simulink model "Comparation_L_and_NL_Lat"  (R2025b)
settings: Solver=ode4  StartTime=0.0  StopTime=10  FixedStep=1/10  RelTol=1e-3
values from neighbouring files (symbols this model uses):
  sys_lat = ss(A_lat, B_lat, C_lat, D_lat,      'StateName',{'beta';'p';'r';'phi';'psi'},      'InputName',{'aileron';'rudder'},      'OutputName',{'beta';'p';'r';'phi';'psi'})    [MATRIZES_DH.m]    (also in modelo_linear_DH.m = ss(A_lat, B_lat, C_lat, D_lat,      'StateName', {'beta'; 'p)
  Ue = [0.283590235022 0.133002178957 0 0 0 0 0]'    [MATRIZES_DH.m]
undefined symbols (not defined in the file or in its folder): sigbuilder_block
settings Model: Creator=anade  LastModifiedBy=mirko

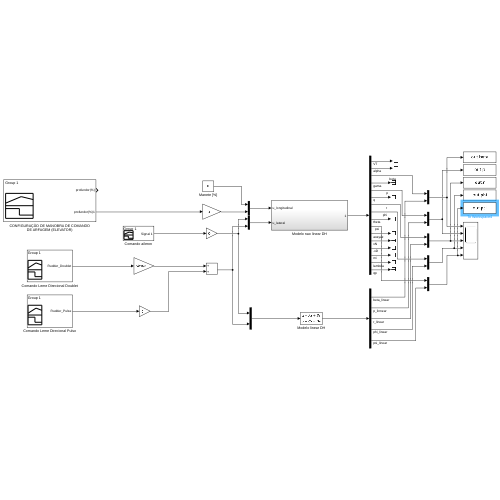
[thumbnail: Simulink's stored preview of the top-level diagram]
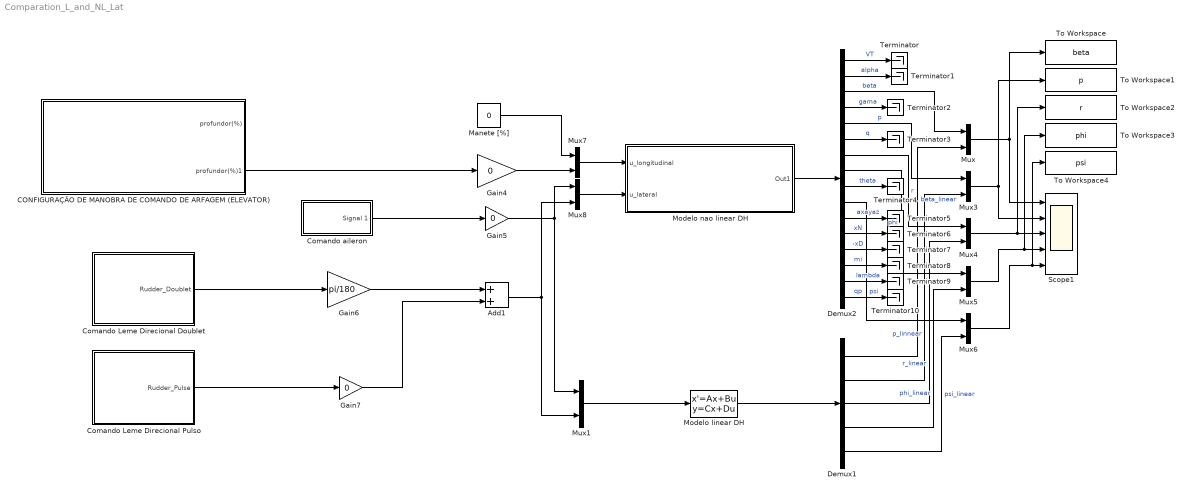
== system Comparation_L_and_NL_Lat ==
  Add1 : Sum
  CONFIGURAÇÃO DE MANOBRA DE COMANDO DE ARFAGEM (ELEVATOR) : Subsystem  Tag=STV Subsys  LoadFcn=sigbuilder_block('load');  StartFcn=sigbuilder_block('start');  StopFcn=sigbuilder_block('stop');  ClipboardFcn=sigbuilder_block('clipboard');  mask(Sigbuilder block){tuvar=[0:10]}
      mask help: Simulink:masks:SigbuilderBlock_MD
      mask init:
      | if ~strcmp(get_param(bdroot(gcbh),'SimulationStatus'),'stopped') tuvar = sigbuilder_block('maskInit'); end
      settings: CopyFcn=sigbuilder_block('copy');  DeleteFcn=sigbuilder_block('delete');  ModelCloseFcn=sigbuilder_block('modelClose');  PreSaveFcn=sigbuilder_block('preSave');  PauseFcn=sigbuilder_block('pause');  ContinueFcn=sigbuilder_block('continue');  NameChangeFcn=sigbuilder_block('namechange');  OpenFcn=sigbuilder_block('open',[437.6 199.2 550.4 400 ]);  CloseFcn=sigbuilder_block('close');
      mask Display: plot(0, 0, 100, 100,[2, 2, 32, 32, 2], [68, 8, 8, 68, 68],[32, 2], [38, 38], [32, 19, 2],[53, 60, 44], [32, 17, 17, 2],[16, 16, 31, 31]);txt = getActiveGroup(gcbh);text(2, 100, txt,'verticalAlignment', 'top');
  Comando Leme Direcional Doublet : Subsystem  Tag=STV Subsys  LoadFcn=sigbuilder_block('load');  StartFcn=sigbuilder_block('start');  StopFcn=sigbuilder_block('stop');  ClipboardFcn=sigbuilder_block('clipboard');  mask(Sigbuilder block){tuvar=[0:10]}
      mask help: Simulink:masks:SigbuilderBlock_MD
      mask init:
      | if ~strcmp(get_param(bdroot(gcbh),'SimulationStatus'),'stopped') tuvar = sigbuilder_block('maskInit'); end
      settings: CopyFcn=sigbuilder_block('copy');  DeleteFcn=sigbuilder_block('delete');  ModelCloseFcn=sigbuilder_block('modelClose');  PreSaveFcn=sigbuilder_block('preSave');  PauseFcn=sigbuilder_block('pause');  ContinueFcn=sigbuilder_block('continue');  NameChangeFcn=sigbuilder_block('namechange');  OpenFcn=sigbuilder_block('open',[316.5 171.75 805.5 485.25 ]);  CloseFcn=sigbuilder_block('close');
      mask Display: plot(0, 0, 100, 100,[2, 2, 32, 32, 2], [68, 8, 8, 68, 68],[32, 2], [38, 38], [32, 19, 2],[53, 60, 44], [32, 17, 17, 2],[16, 16, 31, 31]);txt = getActiveGroup(gcbh);text(2, 100, txt,'verticalAlignment', 'top');
  Comando Leme Direcional Pulso : Subsystem  Tag=STV Subsys  LoadFcn=sigbuilder_block('load');  StartFcn=sigbuilder_block('start');  StopFcn=sigbuilder_block('stop');  ClipboardFcn=sigbuilder_block('clipboard');  mask(Sigbuilder block){tuvar=[0:10]}
      mask help: Simulink:masks:SigbuilderBlock_MD
      mask init:
      | if ~strcmp(get_param(bdroot(gcbh),'SimulationStatus'),'stopped') tuvar = sigbuilder_block('maskInit'); end
      settings: CopyFcn=sigbuilder_block('copy');  DeleteFcn=sigbuilder_block('delete');  ModelCloseFcn=sigbuilder_block('modelClose');  PreSaveFcn=sigbuilder_block('preSave');  PauseFcn=sigbuilder_block('pause');  ContinueFcn=sigbuilder_block('continue');  NameChangeFcn=sigbuilder_block('namechange');  OpenFcn=sigbuilder_block('open',[463.8 78 543 376.2 ]);  CloseFcn=sigbuilder_block('close');
      mask Display: plot(0, 0, 100, 100,[2, 2, 32, 32, 2], [68, 8, 8, 68, 68],[32, 2], [38, 38], [32, 19, 2],[53, 60, 44], [32, 17, 17, 2],[16, 16, 31, 31]);txt = getActiveGroup(gcbh);text(2, 100, txt,'verticalAlignment', 'top');
  Comando aileron : Subsystem  Tag=STV Subsys  LoadFcn=sigbuilder_block('load');  StartFcn=sigbuilder_block('start');  StopFcn=sigbuilder_block('stop');  ClipboardFcn=sigbuilder_block('clipboard');  mask(Sigbuilder block){tuvar=[0:10]}
      mask help: Simulink:masks:SigbuilderBlock_MD
      mask init:
      | if ~strcmp(get_param(bdroot(gcbh),'SimulationStatus'),'stopped') tuvar = sigbuilder_block('maskInit'); end
      settings: CopyFcn=sigbuilder_block('copy');  DeleteFcn=sigbuilder_block('delete');  ModelCloseFcn=sigbuilder_block('modelClose');  PreSaveFcn=sigbuilder_block('preSave');  PauseFcn=sigbuilder_block('pause');  ContinueFcn=sigbuilder_block('continue');  NameChangeFcn=sigbuilder_block('namechange');  OpenFcn=sigbuilder_block('open',[6.75 6.75 1134.75 568.5 ]);  CloseFcn=sigbuilder_block('close');
      mask Display: plot(0, 0, 100, 100,[2, 2, 32, 32, 2], [68, 8, 8, 68, 68],[32, 2], [38, 38], [32, 19, 2],[53, 60, 44], [32, 17, 17, 2],[16, 16, 31, 31]);txt = getActiveGroup(gcbh);text(2, 100, txt,'verticalAlignment', 'top');
  Demux1 : Demux  Outputs=5
  Demux2 : Demux  Outputs=16
  Gain4 : Gain  Gain=0  OutDataTypeStr=double
  Gain5 : Gain  Gain=0
  Gain6 : Gain  Gain=pi/180
  Gain7 : Gain  Gain=0
  Manete [%] : Constant  Value=0
  Modelo linear DH : StateSpace  A=sys_lat.A  B=sys_lat.B  C=sys_lat.C  D=sys_lat.D  InitialCondition=[0 0 0 0 0]
  Modelo nao linear DH : Subsystem
  Mux{,1,3..8} (8 alike) : Mux  Inputs=2
  Scope1 : Scope  NumInputPorts=5
      settings: ActiveDisplayYMinimum=-4.5855532586935484  ActiveDisplayYMaximum=3.8994861451279332
  Terminator{,1..10} (11 alike) : Terminator
  To Workspace : ToWorkspace  VariableName=beta  SaveFormat=Structure With Time  SampleTime=-1
  To Workspace1 : ToWorkspace  VariableName=p  SaveFormat=Structure With Time  SampleTime=-1
  To Workspace2 : ToWorkspace  VariableName=r  SaveFormat=Structure With Time  SampleTime=-1
  To Workspace3 : ToWorkspace  VariableName=phi  SaveFormat=Structure With Time  SampleTime=-1
  To Workspace4 : ToWorkspace  VariableName=psi  SaveFormat=Structure With Time  SampleTime=-1
  wires:
  Mux1/1 -> Modelo linear DH/1
  Modelo linear DH/1 -> Demux1/1
  Mux/1 -> To Workspace/1, Scope1/1
  Demux1/2 -> Mux3/2  "p_linnear"
  Demux1/3 -> Mux4/2  "r_linear"
  Demux1/4 -> Mux5/2  "phi_linear"
  Demux1/5 -> Mux6/2  "psi_linear"
  Mux3/1 -> To Workspace1/1, Scope1/2
  Mux4/1 -> Scope1/3, To Workspace2/1
  Mux5/1 -> To Workspace3/1, Scope1/4
  Mux6/1 -> To Workspace4/1, Scope1/5
  Demux1/1 -> Mux/2  "beta_linear"
  Mux7/1 -> Modelo nao linear DH/1(u_longitudinal)
  Gain7/1 -> Add1/2
  Comando Leme Direcional Pulso/1(Rudder_Pulse) -> Gain7/1
  Modelo nao linear DH/1(Out1) -> Demux2/1
  Gain5/1 -> Mux8/1, Mux1/1
  Comando Leme Direcional Doublet/1(Rudder_Doublet) -> Gain6/1
  Demux2/3 -> Mux/1  "beta"
  Gain4/1 -> Mux7/2
  Comando aileron/1(Signal 1) -> Gain5/1
  Demux2/10 -> Mux6/1  "psi"
  Demux2/5 -> Mux3/1  "p"
  Gain6/1 -> Add1/1
  Demux2/8 -> Mux5/1  "phi"
  CONFIGURAÇÃO DE MANOBRA DE COMANDO DE ARFAGEM (ELEVATOR)/2(profundor(%)1) -> Gain4/1
  Mux8/1 -> Modelo nao linear DH/2(u_lateral)
  Demux2/7 -> Mux4/1  "r"
  Add1/1 -> Mux8/2, Mux1/2
  Manete [%]/1 -> Mux7/1
  Demux2/1 -> Terminator/1  "VT"
  Demux2/2 -> Terminator1/1  "alpha"
  Demux2/4 -> Terminator2/1  "gama"
  Demux2/6 -> Terminator3/1  "q"
  Demux2/9 -> Terminator4/1  "theta"
  Demux2/11 -> Terminator5/1  "axayaz"
  Demux2/12 -> Terminator6/1  "xN"
  Demux2/13 -> Terminator7/1  "-xD"
  Demux2/14 -> Terminator8/1  "mi"
  Demux2/15 -> Terminator9/1  "lambda"
  Demux2/16 -> Terminator10/1  "qp"

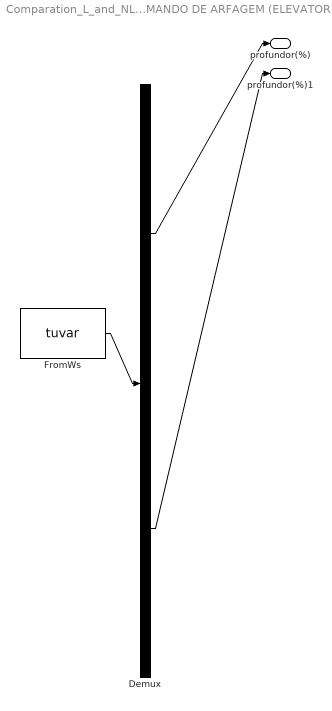
== system Comparation_L_and_NL_Lat/CONFIGURAÇÃO DE MANOBRA DE COMANDO DE ARFAGEM (ELEVATOR) ==
  Demux : Demux  Tag=STV Demux  Outputs=2
      settings: DisplayOption=none
  FromWs : FromWorkspace  Tag=STV FromWs  VariableName=tuvar
      SigBuilderData=|
      | common.afterFinalStr = 'Extrapolate'
      | common.sampleTime = '0'
      | dataSet.timeRange = [0 100]
      | dataSet.name = 'Group 1'
      | sbobj.Groups.Name = 'Group 1'
      | sbobj.Groups.Signals(1).Name = 'profundor(%)'
      | sbobj.Groups.Signals(1).XData = [0 0.1 0.2 0.3 0.4 0.5 0.6 0.7 0.8 0.9 1 1.1 1.2 1.3 1.4 1.5 1.6 1.7 1.8 1.9 2 2.1 2.2 2.3 2.4 2.5 2.6 2.7 2.8 2.9 3 3.1 3.2 3.3 3.4 3.5 3.6 3.7 3.8 3.9 4 4.1 4.2 4.3 4.4 4.5 4.6 4.7 4.8 4.9 5 5.1 5.2 5.3 5.4 5.5 5.6 5.7 5.8 5.9 6 6.1 6.2 6.3 6.4 6.5 6.6 6.7 6.8 6.9 7 7.1 7.2 7.3 7.4 7.5 7.6 7.7 7.8 7.9 8 8.1 8.2 8.3 8.4 8.5 8.6 8.7 8.8 8.9 9 9.1 9.2 9.3 9.4 9.5 9.6 9.7 9.8 100]
      | sbobj.Groups.Signals(1).YData = [0 0 0 0 0 0 0 0.00760496509518 0.0155943823498 0 0 0 -0.00125864493304 -0.0124354709205 0 0 0 0.001308996939 0.0121726919983 0 0 0 0.19836946068 0.26049039086 0.0145934241644 -0.242818932184 -0.18442905898 -0.00242557317913 0.00517884512025 -0.000654498469498 -0.000654498469498 -0.000654498469498 -0.000654498469498 -0.000654498469498 -0.000654498469498 -0.000654498469498 -0.000654498469498 -0.000654498469498 -0.000654498469498 -0.000654498469498 -0.000654498469498 -0.000654498469498 -0.000654498469498 -0.000654498469498 -0.000654498469498 -0.000654498469498 -0.000654498469498 -0.000654498469498 -0.000654498469498 -0.000654498469498 -0.000654498469498 -0.000654498469498 -0.000654498469498 -0.000654498469498 -0.000654498469498 -0.000654498469498 -0.000654498469498 -0.000654498469498 -0.000654498469498 -0.000654498469498 -0.000654498469498 -0.000654498469498 -0.000654498469498 -0.000654498469498 -0.000654498469498 -0.000654498469498 -0.000654498469498 -0.000654498469498 -0.000654498469498 -0.000654498469498 -0.000654498469498 -0.000654498469498 -0.000654498469498 -0.000654498469498 -0.000654498469498 -0.000654498469498 -0.000654498469498 -0.000654498469498 -0.000654498469498 -0.000654498469498 -0.000654498469498 -0.000654498469498 -0.000654498469498 -0.000654498469498 -0.000654498469498 -0.000654498469498 -0.000654498469498 -0.000654498469498 -0.000654498469498 -0.000654498469498 -0.000654498469498 -0.000654498469498 -0.000654498469498 -0.000654498469498 -0.000654498469498 -0.000654498469498 -0.000654498469498 -0.000654498469498 -0.000654498469498 -0.000654498469498]
      | sbobj.Groups.Signals(2).Name = 'profundor(%)1'
      | sbobj.Groups.Signals(2).XData = [0 0.1 0.2 0.3 0.4 0.5 0.6 0.7 0.8 0.9 1 1.1 1.2 1.3 1.4 1.5 1.6 1.7 1.8 1.9 2 2.1 2.2 2.3 2.4 2.5 2.6 2.7 2.8 2.9 3 3.1 3.2 3.3 3.4 3.5 3.6 3.7 3.8 3.9 4 4.1 4.2 4.3 4.4 4.5 4.6 4.7 4.8 4.9 5 5.1 5.2 5.3 5.4 5.5 5.6 5.7 5.8 5.9 6 6.1 6.2 6.3 6.4 6.5 6.6 6.7 6.8 6.9 7 7.1 7.2 7.3 7.4 7.5 7.6 7.7 7.8 7.9 8 8.1 8.2 8.3 8.4 8.5 8.6 8.7 8.8 8.9 9 9.1 9.2 9.3 9.4 9.5 9.6 9.7 9.8 9.9 100]
      | sbobj.Groups.Signals(2).YData = [-0.00659899366307 -0.00196349540849 -0.00196349540849 -0.00196349540849 -0.00196349540849 -0.00196349540849 -0.00196349540849 -0.00196349540849 -0.00196349540849 -0.00196349540849 -0.00196349540849 -0.00196349540849 -0.00196349540849 -0.00196349540849 -0.000981456676208 0.0111264739815 0 0 0 0 0.00816755750239 0.116620098461 0.252914916546 0.0615228561328 -0.242128079656 -0.0902454404262 0.0467302060423 -0.0124354709205 0 0 0 0 0 0 0 0 0 0 0 0 0 0 0 0 0 0 0 0 0 0 0 0 0 0 0 0 0 0 0 0 0 0 0 0 0 0 0 0 0 0 0 0 0 0 0 0 0 0 0 0 0 0 0 0 0 0 0 0 0 0 0 0 0 0 0 0 0 0 0 0.001308996939 0.001308996939]
      | sbobj.Groups.TimeRange = [0 100]
  profundor(%) : Outport  Tag=STV Outport
  profundor(%)1 : Outport  Tag=STV Outport  Port=2
  wires:
  FromWs/1 -> Demux/1
  Demux/1 -> profundor(%)/1
  Demux/2 -> profundor(%)1/1

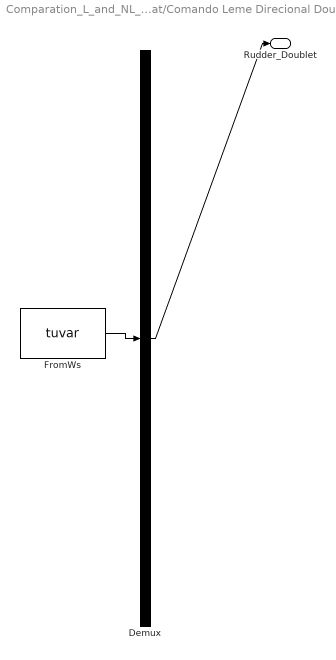
== system Comparation_L_and_NL_Lat/Comando Leme Direcional Doublet ==
  Demux : Demux  Tag=STV Demux  Outputs=1
      settings: DisplayOption=none
  FromWs : FromWorkspace  Tag=STV FromWs  VariableName=tuvar
      SigBuilderData=|
      | common.afterFinalStr = 'Extrapolate'
      | common.sampleTime = 0
      | dataSet.timeRange = [0 1000]
      | dataSet.name = 'Group 1'
      | sbobj.Groups.Name = 'Group 1'
      | sbobj.Groups.Signals.Name = 'Rudder_Doublet'
      | sbobj.Groups.Signals.XData = [0 4 4 4.36 4.36 4.86 4.86 1000]
      | sbobj.Groups.Signals.YData = [0 0 10 10 -10.2 -10.2 0 0]
      | sbobj.Groups.TimeRange = [0 1000]
  Rudder_Doublet : Outport  Tag=STV Outport
  wires:
  FromWs/1 -> Demux/1
  Demux/1 -> Rudder_Doublet/1

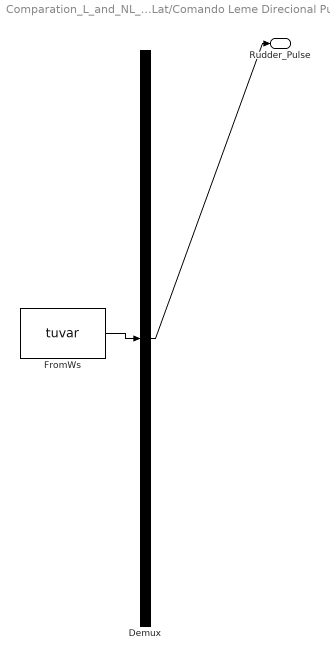
== system Comparation_L_and_NL_Lat/Comando Leme Direcional Pulso ==
  Demux : Demux  Tag=STV Demux  Outputs=1
      settings: DisplayOption=none
  FromWs : FromWorkspace  Tag=STV FromWs  VariableName=tuvar
      SigBuilderData=|
      | common.afterFinalStr = 'Extrapolate'
      | common.sampleTime = 0
      | dataSet.timeRange = [0 1000]
      | dataSet.name = 'Group 1'
      | sbobj.Groups.Name = 'Group 1'
      | sbobj.Groups.Signals.Name = 'Rudder_Pulse'
      | sbobj.Groups.Signals.XData = [0 4 4 7.2 7.2 1000]
      | sbobj.Groups.Signals.YData = [0 0 10 10 -2e-05 -2e-05]
      | sbobj.Groups.TimeRange = [0 1000]
  Rudder_Pulse : Outport  Tag=STV Outport
  wires:
  FromWs/1 -> Demux/1
  Demux/1 -> Rudder_Pulse/1

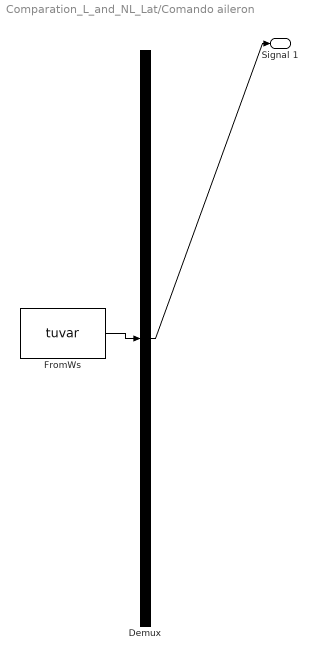
== system Comparation_L_and_NL_Lat/Comando aileron ==
  Demux : Demux  Tag=STV Demux  Outputs=1
      settings: DisplayOption=none
  FromWs : FromWorkspace  Tag=STV FromWs  VariableName=tuvar
      SigBuilderData=|
      | common.afterFinalStr = 'Extrapolate'
      | common.sampleTime = 0
      | dataSet.timeRange = [0 1000]
      | dataSet.name = 'Group 1'
      | sbobj.Groups.Name = 'Group 1'
      | sbobj.Groups.Signals.Name = 'Signal 1'
      | sbobj.Groups.Signals.XData = [0 4.95 4.95 7 7 1000]
      | sbobj.Groups.Signals.YData = [0 0 1.005 1.005 0 0]
      | sbobj.Groups.TimeRange = [0 1000]
  Signal 1 : Outport  Tag=STV Outport
  wires:
  FromWs/1 -> Demux/1
  Demux/1 -> Signal 1/1

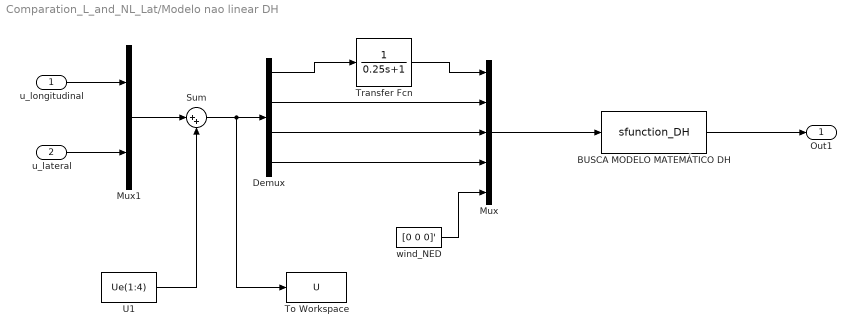
== system Comparation_L_and_NL_Lat/Modelo nao linear DH ==
  u_longitudinal : Inport
  u_lateral : Inport  Port=2
  "BUSCA MODELO MATEMÁTICO DH " : S-Function  FunctionName=sfunction_DH  Parameters=Xe, coef_Sato, coef_Ana  SFunctionDeploymentMode=off  EnableBusSupport=off
  Demux : Demux
  Mux : Mux  Inputs=5
  Mux1 : Mux  Inputs=2
  Sum : Sum  Inputs=|++
  To Workspace : ToWorkspace  VariableName=U  SampleTime=-1
  Transfer Fcn : TransferFcn  Denominator=[0.25 1]
  U1 : Constant  Value=Ue(1:4)
  wind_NED : Constant  Value=[0 0 0]'
  Out1 : Outport
  wires:
  wind_NED/1 -> Mux/5
  u_longitudinal/1 -> Mux1/1
  u_lateral/1 -> Mux1/2
  U1/1 -> Sum/2
  Sum/1 -> Demux/1, To Workspace/1
  Mux1/1 -> Sum/1
  Mux/1 -> "BUSCA MODELO MATEMÁTICO DH "/1
  Demux/1 -> Transfer Fcn/1
  Demux/2 -> Mux/2
  Demux/3 -> Mux/3
  Demux/4 -> Mux/4
  "BUSCA MODELO MATEMÁTICO DH "/1 -> Out1/1
  Transfer Fcn/1 -> Mux/1
